simulink model "drymodel"  (R2020b)
settings: Solver=ode45  StartTime=0.0  StopTime=inf  RelTol=1e-3  EnableMultiTasking=on
values from neighbouring files (symbols this model uses):
  s = evalin('base','s')    [GUI_MT44001.m]
undefined symbols (not defined in the file or in its folder): TS_boat
libraries: simulink x5
settings Model: Creator=Andries  LastModifiedBy=LocalAdmin
settings DataIOCC: LimitDataPoints=on  SaveFormat=Array  SignalLoggingSaveFormat=ModelDataLogs  ReturnWorkspaceOutputs=off
settings OptimizationCC: ExpressionDepthLimit=2147483647  LifeSpan=inf
settings DebuggingCC: UnderspecifiedInitializationDetection=Classic  MergeDetectMultiDrivingBlocksExec=none  SolverPrmCheckMsg=warning  FcnCallInpInsideContextMsg=warning  StateNameClashWarn=warning  SFUnexpectedBacktrackingDiag=warning  SFNoUnconditionalDefaultTransitionDiag=warning  SFExecutionAtInitializationDiag=none  ArithmeticOperatorsInVariantConditions=warning
settings HardwareCC: ProdBitPerPointer=32  ProdBitPerSizeT=32  ProdBitPerPtrDiffT=32  ProdLargestAtomicFloat=None  ProdIntDivRoundTo=Undefined  ProdEndianess=Unspecified  ProdWordSize=32  ProdHWDeviceType=32-bit Generic
settings ModelReferenceCC: PropagateSignalLabelsOutOfModel=off
settings SFSimCC: SimUseLocalCustomCode=off  CustomCodeUndefinedFunction=UseInterfaceOnly
settings RTWCC: RTWUseLocalCustomCode=off
settings CodeAppCC: StateflowObjectComments=on
settings GRTTargetCC: TargetLangStandard=C89/C90 (ANSI)  CombineOutputUpdateFcns=off  GRTInterface=on
settings ConfigComp: CovMetricSettings=dw  CovSaveCumulativeToWorkspaceVar=on  CovSaveSingleToWorkspaceVar=on  CovExternalEMLEnable=off

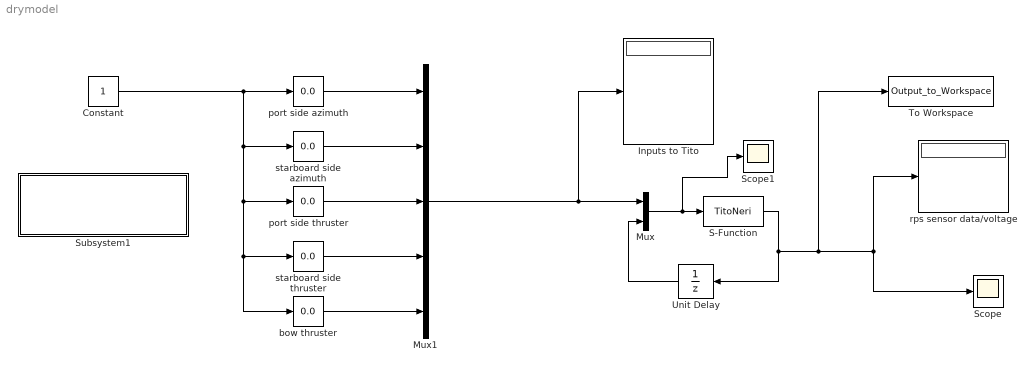
== system drymodel ==
  Constant : Constant
  Inputs to Tito : Display
  Mux : Mux  Inputs=2
  Mux1 : Mux  Inputs=5
  S-Function : S-Function  FunctionName=TitoNeri  Parameters=TS_boat,s  SFunctionDeploymentMode=off  EnableBusSupport=off
  Scope : Scope
  Scope1 : Scope
  Subsystem1 : Subsystem
      mask Display:
      | if evalin('base','exist(''boat'')');
      |     set_param(gcb,'BackgroundColor','Green')
      |     disp(['connected to: ',evalin('base','boat.name')]);
      | else
      |     disp('no boat connected')
      |     set_param(gcb,'BackgroundColor','Red')
      |     color('red')
      | end
  To Workspace : ToWorkspace  VariableName=Output_to_Workspace  SampleTime=-1
  Unit Delay : UnitDelay  SampleTime=-1  HasFrameUpgradeWarning=on
  bow thruster : simulink/Math Operations/Slider Gain  gain=0.0  low=-0.4  high=0.4
  port side azimuth : simulink/Math Operations/Slider Gain  gain=0.0  low=-1  high=1
  port side thruster : simulink/Math Operations/Slider Gain  gain=0.0  low=-1  high=1
  rps sensor data/voltage : Display
  starboard side azimuth : simulink/Math Operations/Slider Gain  gain=0.0  low=-1  high=1
  starboard side thruster : simulink/Math Operations/Slider Gain  gain=0.0  low=-1  high=1
  wires:
  Constant/1 -> port side azimuth/1, starboard side azimuth/1, port side thruster/1, starboard side thruster/1, bow thruster/1
  port side azimuth/1 -> Mux1/1
  starboard side azimuth/1 -> Mux1/2
  port side thruster/1 -> Mux1/3
  starboard side thruster/1 -> Mux1/4
  bow thruster/1 -> Mux1/5
  Mux1/1 -> Mux/1, Inputs to Tito/1
  Mux/1 -> Scope1/1, S-Function/1
  Unit Delay/1 -> Mux/2
  S-Function/1 -> Unit Delay/1, To Workspace/1, rps sensor data/voltage/1, Scope/1

== system drymodel/Subsystem1 ==
